simulink model "playback_data_4"  (R2015a)
settings: Solver=FixedStepDiscrete  SolverMode=SingleTasking  StartTime=0  StopTime=time_recorded(end)  FixedStep=sample_time  RelTol=1e-3
undefined symbols (not defined in the file): A1_notch_f1, A2_notch_f1, A_kalman_transverse, A_kalman_vertical, A_lpf_dtau, A_lpf_fourbar_angles, A_lpf_imu, A_lpf_lateral_angle, A_lpf_leg_spring, B1_lpf_dtau, B1_lpf_fourbar_angles, B1_lpf_imu, B1_lpf_lateral_angle, B1_lpf_leg_spring, B1_notch_f1, B2_lpf_dtau, B2_lpf_fourbar_angles, B2_lpf_imu, B2_lpf_lateral_angle, B2_lpf_leg_spring, B2_notch_f1, B_dx_versus_x0, B_kalman_transverse, B_kalman_vertical, backwards_K_front_of_t_row1, backwards_K_front_of_t_row2, backwards_K_sag_of_t, backwards_P_front_of_t, backwards_P_sag_of_t, C_kalman_transverse, C_kalman_vertical, com_leg_motor, com_torso, contact_threshold, control_start_time, d_ankle_to_foot, d_vertical_com, desired_com_forward_velocity, desired_com_lateral_velocity, desired_initial_leg_roll_left, desired_initial_leg_roll_right, desired_lateral_symmetry_angle, desired_standing_torso_pitch, desired_standing_torso_roll, desired_standing_z, desired_torso_pitch, desired_torso_roll, Discrete, fcut_contact, forward_dx_of_dxstar, forward_x_of_dxstar, g, gain_nodes_sea_torque, HIP_MTR_MAX_CONT_TORQUE, HIP_MTR_MAX_TORQUE, i_leg_motor, i_robot, i_torso, initial_dx_estimate, initial_dy_estimate ... (+75)
libraries: simulink x12, ctrlSharedLib x3
(part 3 of 5)

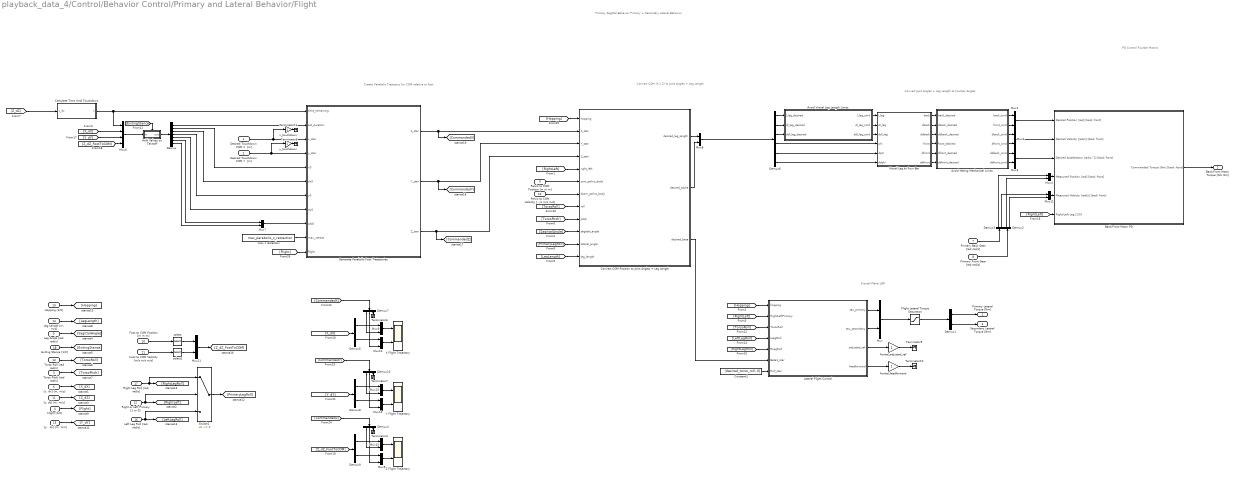
== system playback_data_4/Control/Behavior Control/Primary and Lateral Behavior/Flight ==
  note: Frontal Plane LQR
  note: PD Control Fourbar Motors
  note: Convert Joint Angles + Leg Length
      | to Fourbar Angles
  note: Convert COM (X,Y,Z) to
      | Joint Angles + Leg Length
  note: Create Parabolic
      | Trajectory for COM relative to foot
  note: Primary Sagittal Behavior
      | Primary + Secondary Lateral Behavior
  Desired Touchdown COM X  [m] : Inport
  Desired Touchdown COM Y  [m] : Inport  Port=2
  Torso Pitch [rad rad/s] : Inport  Port=3
  Flight [1/0] : Inport  Port=4
  Leg Angle [rad rad/s] : Inport  Port=5
  "[x, dx] [m, m/s]" : Inport  Port=6
  Primary Back Gear [rad rad/s] : Inport  Port=7
  Primary Front Gear [rad rad/s] : Inport  Port=8
  Pelvis to COM Position [m m m] : Inport  Port=9
  Pelvis to COM Velocity [m/s m/s m/s] : Inport  Port=10
  "[z, dz] [m, m/s]" : Inport  Port=11
  Right or Left Primary [1 or 0] : Inport  Port=12
  Torso Roll [rad rad/s] : Inport  Port=13
  "Leg Length [m, m/s]" : Inport  Port=14
  "[y,  dy] [m, m/s]" : Inport  Port=15
  "Left Leg Roll [rad, rad/s]" : Inport  Port=16
  "Right Leg Roll [rad, rad/s]" : Inport  Port=17
  Exiting Stance [1/0] : Inport  Port=18
  Hopping [1/0] : Inport  Port=19
  Foot to COM Position [m m m] : Inport  Port=20
  Foot to COM Velocity [m/s m/s m/s] : Inport  Port=21
  Avoid Hitting Mechanical Limits : MATLAB Function  TreatAsAtomicUnit=on
  Avoid Virtual Leg Length Limits : MATLAB Function  TreatAsAtomicUnit=on
  Back/Front Motor PD : Subsystem
  Calculate Time Until Touchdown : MATLAB Function  TreatAsAtomicUnit=on
  Constant1 : Constant  Value=[desired_torso_roll; 0]
  "Convert COM Position to Joint Angles + Leg Length " : MATLAB Function  TreatAsAtomicUnit=on
  Demux : Demux  Outputs=7
  Demux{1..3,5,8..9} (6 alike) : Demux  Outputs=2
  Demux10 : Demux  Outputs=3
  Demux4 : Demux  Outputs=3
  Demux6 : Demux  Outputs=6
  Demux7 : Demux  Outputs=3
  Flight Lateral Torque Saturation : Saturate  UpperLimit=HIP_MTR_MAX_CONT_TORQUE  LowerLimit=-HIP_MTR_MAX_CONT_TORQUE
      settings: AttributesFormatString=Top: %<UpperLimit>\nBottom: %<LowerLimit>
  Generate Parabolic Foot Trajectories : MATLAB Function  TreatAsAtomicUnit=on
  Hold Values on Takeoff : Subsystem
  Lateral Flight Control : MATLAB Function  TreatAsAtomicUnit=on
  Mux{,1..5,7..13,15,21} (15 alike) : Mux  Inputs=2
  Mux6 : Mux
  Switch1 : Switch  Criteria=u2 ~= 0
  Terminator{4..7,9..11} (7 alike) : Terminator
  Virtual Leg to Four Bar : MATLAB Function  TreatAsAtomicUnit=on
  X Flight Trajectory : Scope  NumInputPorts=2
      settings: YMin=-1~-0.8  YMax=1~1.4  SaveName=ScopeData3  SampleInput=on
  Y Flight Trajectory : Scope  NumInputPorts=2
      settings: YMin=-1~-0.8  YMax=1~1.4  SaveName=ScopeData4  SampleInput=on
  Z Flight Trajectory : Scope  NumInputPorts=2
      settings: YMin=-1~-0.8  YMax=1~1.4  SaveName=ScopeData7  SampleInput=on
  frontal_adjusted_ref : Gain
  frontal_feedforward : Gain
  max z retraction : Constant  Value=max_parabolic_z_retraction
  select : Selector  InputPortWidth=3  Indices=[3]
  select1 : Selector  InputPortWidth=3  Indices=[3]
  x_touchdown : Gain
  y_touchdown : Gain
  Back/Front Motor Torque [Nm Nm] : Outport
  Primary Lateral Torque [Nm] : Outport  Port=2
  Secondary Lateral Torque [Nm] : Outport  Port=3
  wires:
  Generate Parabolic Foot Trajectories/3(Z_star) -> [CommandedZ], "Convert COM Position to Joint Angles + Leg Length "/4(Z_star)
  [CommandedZ] -> Demux4/1
  [CommandedY] -> Demux10/1
  [CommandedX] -> Demux7/1
  Demux10/3 -> Terminator7/1
  [Y_dY] -> Demux8/1
  Demux10/2 -> Mux12/2
  Demux10/1 -> Mux13/2
  Demux8/2 -> Mux12/1
  Demux8/1 -> Mux13/1
  Mux12/1 -> Y Flight Trajectory/2
  Mux13/1 -> Y Flight Trajectory/1
  Demux7/3 -> Terminator6/1
  [X_dX] -> Demux5/1
  Demux7/2 -> Mux10/2
  Demux7/1 -> Mux9/2
  Demux5/2 -> Mux10/1
  Demux5/1 -> Mux9/1
  Mux10/1 -> X Flight Trajectory/2
  Mux9/1 -> X Flight Trajectory/1
  Demux4/3 -> Terminator4/1
  Demux4/2 -> Mux5/2
  Demux4/1 -> Mux15/2
  Demux9/2 -> Mux5/1
  Demux9/1 -> Mux15/1
  [Z_dZ_FootToCOM] -> Demux9/1
  [Z_dZ_FootToCOM] -> Mux6/4
  Mux5/1 -> Z Flight Trajectory/2
  Mux15/1 -> Z Flight Trajectory/1
  Mux21/1 -> [Z_dZ_FootToCOM]
  select1/1 -> Mux21/2
  select/1 -> Mux21/1
  Foot to COM Velocity [m/s m/s m/s]/1 -> select1/1
  Foot to COM Position [m m m]/1 -> select/1
  Demux/7 -> Mux7/2
  Demux/6 -> Mux7/1
  Demux/5 -> Generate Parabolic Foot Trajectories/8(dy0)
  Demux/4 -> Generate Parabolic Foot Trajectories/7(y0)
  Demux/3 -> Generate Parabolic Foot Trajectories/6(dx0)
  Demux/2 -> Generate Parabolic Foot Trajectories/5(x0)
  [Flight] -> Generate Parabolic Foot Trajectories/11(flight)
  Hopping [1/0]/1 -> [Hopping]
  [Hopping] -> Lateral Flight Control/1(hopping)
  Mux/1 -> Flight Lateral Torque Saturation/1
  [Hopping] -> "Convert COM Position to Joint Angles + Leg Length "/1(hopping)
  frontal_adjusted_ref/1 -> Terminator9/1
  frontal_feedforward/1 -> Terminator10/1
  Flight Lateral Torque Saturation/1 -> Demux1/1
  "Convert COM Position to Joint Angles + Leg Length "/3(desired_beta) -> Lateral Flight Control/6(Beta1_star)
  Demux1/2 -> Secondary Lateral Torque [Nm]/1
  Demux1/1 -> Primary Lateral Torque [Nm]/1
  Exiting Stance [1/0]/1 -> [ExitingStance]
  Switch1/1 -> [PrimaryLegRoll]
  Right or Left Primary [1 or 0]/1 -> [RightLeft], Switch1/2
  "Right Leg Roll [rad, rad/s]"/1 -> [RightLegRoll], Switch1/1
  [RightLegRoll] -> Lateral Flight Control/5(RLegRoll)
  [LeftLegRoll] -> Lateral Flight Control/4(LLegRoll)
  "Left Leg Roll [rad, rad/s]"/1 -> [LeftLegRoll], Switch1/3
  Lateral Flight Control/1(tau_primary) -> Mux/1
  Lateral Flight Control/2(tau_secondary) -> Mux/2
  Lateral Flight Control/4(feedforward) -> frontal_feedforward/1
  Lateral Flight Control/3(adjusted_ref) -> frontal_adjusted_ref/1
  Constant1/1 -> Lateral Flight Control/7(Roll_star)
  [TorsoRoll] -> Lateral Flight Control/3(TorsoRoll)
  [RightLeft] -> Lateral Flight Control/2(RightLeftPrimary)
  Desired Touchdown COM Y  [m]/1 -> Generate Parabolic Foot Trajectories/4(y_star), y_touchdown/1
  Demux6/3 -> Avoid Virtual Leg Length Limits/3(ddl_leg_desired)
  Demux6/2 -> Avoid Virtual Leg Length Limits/2(dl_leg_desired)
  Demux6/1 -> Avoid Virtual Leg Length Limits/1(l_leg_desired)
  Avoid Virtual Leg Length Limits/3(ddl_leg_cmd) -> Virtual Leg to Four Bar/3(ddl_leg)
  Avoid Virtual Leg Length Limits/2(dl_leg_cmd) -> Virtual Leg to Four Bar/2(dl_leg)
  Avoid Virtual Leg Length Limits/1(l_leg_cmd) -> Virtual Leg to Four Bar/1(l_leg)
  Calculate Time Until Touchdown/1(t) -> Generate Parabolic Foot Trajectories/1(time_remaining), Mux6/1
  [Z_dZ] -> Calculate Time Until Touchdown/1(z_dz)
  [Y_dY] -> Mux6/3
  "[y,  dy] [m, m/s]"/1 -> [Y_dY]
  y_touchdown/1 -> Terminator5/1
  x_touchdown/1 -> Terminator11/1
  Desired Touchdown COM X  [m]/1 -> x_touchdown/1, Generate Parabolic Foot Trajectories/3(x_star)
  "[z, dz] [m, m/s]"/1 -> [Z_dZ]
  "Leg Length [m, m/s]"/1 -> [LegLength]
  Torso Roll [rad rad/s]/1 -> [TorsoRoll]
  "[x, dx] [m, m/s]"/1 -> [X_dX]
  [ExitingStance] -> Hold Values on Takeoff/Trigger
  Flight [1/0]/1 -> [Flight]
  Pelvis to COM Velocity [m/s m/s m/s]/1 -> "Convert COM Position to Joint Angles + Leg Length "/7(dcom_pelvis_body)
  Pelvis to COM Position [m m m]/1 -> "Convert COM Position to Joint Angles + Leg Length "/6(com_pelvis_body)
  [TorsoRoll] -> "Convert COM Position to Joint Angles + Leg Length "/8(roll)
  [LegLength] -> "Convert COM Position to Joint Angles + Leg Length "/12(leg_length)
  [PrimaryLegRoll] -> "Convert COM Position to Joint Angles + Leg Length "/11(lateral_angle)
  [TorsoPitch] -> "Convert COM Position to Joint Angles + Leg Length "/9(pitch)
  Torso Pitch [rad rad/s]/1 -> [TorsoPitch]
  [SagittalAngle] -> "Convert COM Position to Joint Angles + Leg Length "/10(sagittal_angle)
  Leg Angle [rad rad/s]/1 -> [SagittalAngle]
  Mux8/1 -> Demux6/1
  Demux6/4 -> Virtual Leg to Four Bar/4(phi)
  Demux6/5 -> Virtual Leg to Four Bar/5(dphi)
  Demux6/6 -> Virtual Leg to Four Bar/6(ddphi)
  "Convert COM Position to Joint Angles + Leg Length "/1(desired_leg_length) -> Mux8/1
  "Convert COM Position to Joint Angles + Leg Length "/2(desired_alpha) -> Mux8/2
  [RightLeft] -> "Convert COM Position to Joint Angles + Leg Length "/5(right_left)
  Generate Parabolic Foot Trajectories/2(Y_star) -> [CommandedY], "Convert COM Position to Joint Angles + Leg Length "/3(Y_star)
  Generate Parabolic Foot Trajectories/1(X_star) -> "Convert COM Position to Joint Angles + Leg Length "/2(X_star), [CommandedX]
  [X_dX] -> Mux6/2
  Hold Values on Takeoff/1(out) -> Demux/1
  Mux6/1 -> Hold Values on Takeoff/1(in)
  max z retraction/1 -> Generate Parabolic Foot Trajectories/10(max_retract)
  Mux7/1 -> Generate Parabolic Foot Trajectories/9(zdz0)
  Demux/1 -> Generate Parabolic Foot Trajectories/2(est_duration)
  [RightLeft] -> Back/Front Motor PD/6(Right/Left Leg [1/0])
  Primary Front Gear [rad rad/s]/1 -> Demux2/1
  Primary Back Gear [rad rad/s]/1 -> Demux3/1
  Back/Front Motor PD/1(Commanded Torque [Nm] [back front]) -> Back/Front Motor Torque [Nm Nm]/1
  Mux3/1 -> Back/Front Motor PD/3(Desired Acceleration [rad/s^2] [back front])
  Mux2/1 -> Back/Front Motor PD/2(Desired Velocity [rad/s] [back front])
  Avoid Hitting Mechanical Limits/6(ddfront_cmd) -> Mux3/2
  Avoid Hitting Mechanical Limits/5(ddback_cmd) -> Mux3/1
  Avoid Hitting Mechanical Limits/4(dfront_cmd) -> Mux2/2
  Avoid Hitting Mechanical Limits/3(dback_cmd) -> Mux2/1
  Demux2/1 -> Mux4/2
  Avoid Hitting Mechanical Limits/1(back_cmd) -> Mux1/1
  Avoid Hitting Mechanical Limits/2(front_cmd) -> Mux1/2
  Demux3/1 -> Mux4/1
  Demux3/2 -> Mux11/1
  Mux1/1 -> Back/Front Motor PD/1(Desired Position [rad] [back front])
  Mux4/1 -> Back/Front Motor PD/4(Measured Position [rad] [back front])
  Demux2/2 -> Mux11/2
  Mux11/1 -> Back/Front Motor PD/5(Measured Velocity [rad/s] [back front])
  Virtual Leg to Four Bar/6(ddfront) -> Avoid Hitting Mechanical Limits/6(ddfront_desired)
  Virtual Leg to Four Bar/5(dfront) -> Avoid Hitting Mechanical Limits/5(dfront_desired)
  Virtual Leg to Four Bar/4(front) -> Avoid Hitting Mechanical Limits/4(front_desired)
  Virtual Leg to Four Bar/3(ddback) -> Avoid Hitting Mechanical Limits/3(ddback_desired)
  Virtual Leg to Four Bar/2(dback) -> Avoid Hitting Mechanical Limits/2(dback_desired)
  Virtual Leg to Four Bar/1(back) -> Avoid Hitting Mechanical Limits/1(back_desired)

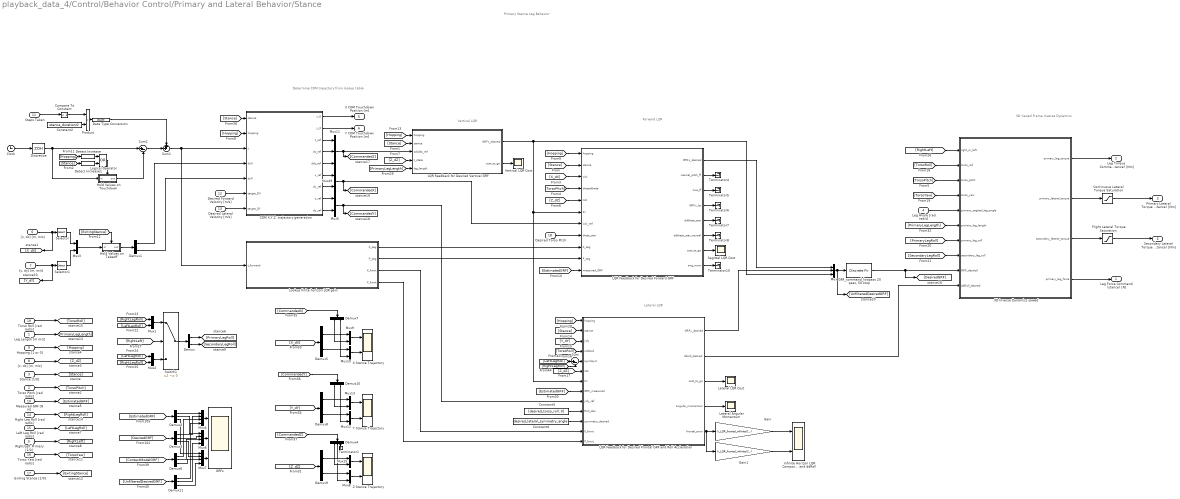
== system playback_data_4/Control/Behavior Control/Primary and Lateral Behavior/Stance ==
  note: Lateral LQR
  note: 3D Yawed Frame Inverse Dynamics
  note: Forward LQR
  note: Vertical LQR
  note: Determine COM trajectory
      | from lookup table
  note: Primary Stance Leg Behavior
  Leg Length [m m/s] : Inport
  Torso Pitch [rad rad/s] : Inport  Port=2
  Stance [1/0] : Inport  Port=3
  Leg Angle [rad rad/s] : Inport  Port=4
  Right/Left Primary [1/0] : Inport  Port=5
  "[x, dx] [m, m/s]" : Inport  Port=6
  "[y, dy] [m, m/s]" : Inport  Port=7
  "[z, dz] [m, m/s]" : Inport  Port=8
  Hopping [1 or 0] : Inport  Port=9
  Measured GRF [N N] : Inport  Port=10
  Steps Taken : Inport  Port=11
  Desired Forward Velocity [m/s] : Inport  Port=12
  Desired Lateral Velocity [m/s] : Inport  Port=13
  Right Leg Roll [rad rad/s] : Inport  Port=14
  Left Leg Roll [rad rad/s] : Inport  Port=15
  Torso Yaw [rad rad/s] : Inport  Port=16
  Exiting Stance [1/0] : Inport  Port=17
  Desired Torso Pitch : Inport  Port=18
  Torso Roll [rad rad/s] : Inport  Port=19
  3D Inverse Dynamics yawed : MATLAB Function  TreatAsAtomicUnit=on
  COM X,Y,Z  trajectory generation : MATLAB Function  TreatAsAtomicUnit=on
  Clock : Clock
  Compare To Constant : simulink/Logic and Bit Operations/Compare To Constant  relop=<  const=1  OutDataTypeStr=uint8
  Constant2 : Constant  Value=stance_duration/2
  Constant5 : Constant  Value=[desired_torso_roll; 0]
  Constant6 : Constant  Value=desired_lateral_symmetry_angle
  Continuous Lateral Torque Saturation : Saturate  UpperLimit=HIP_MTR_MAX_CONT_TORQUE  LowerLimit=-HIP_MTR_MAX_CONT_TORQUE
      settings: AttributesFormatString=Top: %<UpperLimit>\nBottom: %<LowerLimit>
  Data Type Conversion : DataTypeConversion  OutDataTypeStr=double
  Demux{,1,5,7..10} (7 alike) : Demux  Outputs=2
  Demux{2..4,6,11} (5 alike) : Demux  Outputs=3
  Detect Increase : simulink/Logic and Bit Operations/Detect Increase  vinit=0.0  InputProcessing=Inherited  OutDataTypeStr=boolean
  Detect Increase1 : simulink/Logic and Bit Operations/Detect Increase  vinit=0.0  InputProcessing=Inherited  OutDataTypeStr=boolean
  Discretize : ZeroOrderHold  SampleTime=sample_time
  Flight Lateral Torque Saturation : Saturate  UpperLimit=HIP_MTR_MAX_CONT_TORQUE  LowerLimit=-HIP_MTR_MAX_CONT_TORQUE
      settings: AttributesFormatString=Top: %<UpperLimit>\nBottom: %<LowerLimit>
  "GRF_command_lowpass 20 pass, 50 stop" : DiscreteFir  Tag=BlockMethodSubSystem  Coefficients=[-0.0065303670489285049 -0.0039313926403470242 -0.0048630776000435465 -0.0057248908722514107 -0.0064402270401543553 -0.0069124881718239713 -0.0070550751837271126 -0.0067763964248262719 -0.0059955884962007702 -0.0046203515932795149 -0.0026164712407433744 5.5625054243875136e-05 0.0034168828763037565 0.0074322120212943236 0.012066519706809652 0.01722807163822164 0.022817702983514012 0.028694941256765513 0.03470395198526529 0.040669941556379492 0.046421058403681451 0.051764290707578361 0.056533861311620921 0.060562831216546612 0.063716802641316989 0.06588388946005809 0.066985417581438667 0.066985417581438667 0.06588388946005809 0.063716802641316989 0.060562831216546612 0.056533861311620921 0.051764290707578361 0.046421058403681451 0.040669941556379492 0.03470395198526529 0.028694941256765513 0.022817702983514012 0.01722807163822164 0.012066519706809652 0.0074322120212943236 0.0034168828763037565 5.5625054243875136e-05 -0.0026164712407433744 -0.0046203515932795149 -0.0059955884962007702 -0.0067763964248262719 -0.0070550751837271126 -0.0069124881718239713 -0.0064402270401543553 -0.0057248908722514107 -0.0048630776000435465 -0.0039313926403470242 -0.0065303670489285049]  SampleTime=sample_time
  GRFs : Scope  NumInputPorts=3
      settings: TimeRange=0.3720061688053303  YMin=-12.5~-40~0  YMax=15~80~4000  SampleInput=on
  Gain : Gain  Gain=k_LQR_frontal_infinite(1,:)
  Gain1 : Gain  Gain=k_LQR_frontal_infinite(2,:)
  Hold Values on Takeoff : Subsystem
  Hold Values on Touchdown : Subsystem
  "Infinite Horizon LQR Components y, roll, sym, dy, droll, L GRFy and ddRoll" : Scope  NumInputPorts=2
      settings: YMin=-3.5~-5  YMax=4~5  SaveName=ScopeData12  SampleInput=on
  LQR Feedback for Desired Forward GRF : MATLAB Function  TreatAsAtomicUnit=on
  LQR Feedback for Desired Frontal GRF and Roll Accleration : MATLAB Function  TreatAsAtomicUnit=on
  LQR Feedback for Desired Vertical GRF : MATLAB Function  TreatAsAtomicUnit=on
  Lateral Angular Momentum : Scope
      settings: YMin=-3.5  YMax=4  SaveName=ScopeData20  SampleInput=on
  Lateral LQR Cost : Scope
      settings: YMin=100  YMax=240  SaveName=ScopeData9  SampleInput=on
  Logical Operator : Logic  Operator=OR  AllPortsSameDT=off  OutDataTypeStr=boolean
  Lookup finite horizon LQR gain : MATLAB Function  TreatAsAtomicUnit=on
  Mux : Mux  Inputs=3
  Mux{1..3,5,8..10,12..13,15,49} (11 alike) : Mux  Inputs=2
  Mux11 : Mux  Inputs=3
  Mux4 : Mux
  Mux6 : Mux
  Mux7 : Mux
  Product : Product
  Sagittal LQR Cost : Scope
      settings: YMin=22.5  YMax=62.5  SaveName=ScopeData10  SampleInput=on
  Selector : Selector  InputPortWidth=2  Indices=[2]
  Selector1 : Selector  InputPortWidth=2  Indices=[2]
  Sum : Sum  Inputs=|+-
  Sum1 : Sum  Inputs=++|  OutDataTypeStr=double
  Sum2 : Sum  Inputs=|+-
  Switch1 : Switch  Criteria=u2 ~= 0
  Terminator{1,4..8,10} (7 alike) : Terminator
  Vertical LQR Cost : Scope
      settings: YMin=11  YMax=16  SaveName=ScopeData18  SampleInput=on
  X Stance Trajectory : Scope  NumInputPorts=2
      settings: YMin=0~-0.02  YMax=0.005~0.03  SaveName=ScopeData8  SampleInput=on
  Y Stance Trajectory : Scope  NumInputPorts=2
      settings: YMin=0.005~-0.5  YMax=0.1~0.3  SaveName=ScopeData5  SampleInput=on
  Z Stance Trajectory : Scope  NumInputPorts=2
      settings: YMin=0~-1.25  YMax=1.05~1.5  SaveName=ScopeData6  SampleInput=on
  Leg Force Command (stance) [N] : Outport
  Leg Torque Command (stance) [Nm] : Outport  Port=2
  Primary Lateral Torque Command (stance) [Nm] : Outport  Port=3
  Secondary Lateral Torque Command (stance) [Nm] : Outport  Port=4
  X COM Touchdown Position [m] : Outport  Port=5
  Y COM Touchdown Position [m] : Outport  Port=6
  wires:
  Gain1/1 -> "Infinite Horizon LQR Components y, roll, sym, dy, droll, L GRFy and ddRoll"/2
  LQR Feedback for Desired Frontal GRF and Roll Accleration/5(frontal_error) -> Gain/1, Gain1/1
  Gain/1 -> "Infinite Horizon LQR Components y, roll, sym, dy, droll, L GRFy and ddRoll"/1
  Continuous Lateral Torque Saturation/1 -> Primary Lateral Torque Command (stance) [Nm]/1
  3D Inverse Dynamics yawed/3(secondary_lateral_torque) -> Flight Lateral Torque Saturation/1
  3D Inverse Dynamics yawed/2(primary_lateral_torque) -> Continuous Lateral Torque Saturation/1
  Demux11/3 -> Mux7/4
  Demux11/2 -> Mux6/4
  Demux11/1 -> Mux4/4
  [UnfilteredDesiredGRF] -> Demux11/1
  "GRF_command_lowpass 20 pass, 50 stop"/1 -> [DesiredGRF], 3D Inverse Dynamics yawed/9(GRF_desired)
  LQR Feedback for Desired Forward GRF/1(GRFx_desired) -> Mux/1
  Left Leg Roll [rad rad/s]/1 -> [LeftLegRoll]
  Right/Left Primary [1/0]/1 -> [RightLeft]
  [CommandedZ] -> Demux4/1
  [CommandedY] -> Demux10/1
  [CommandedX] -> Demux7/1
  [Y_dY] -> Demux8/1
  Demux10/2 -> Mux12/2
  Demux10/1 -> Mux13/2
  Demux8/2 -> Mux12/1
  Demux8/1 -> Mux13/1
  Mux12/1 -> Y Stance Trajectory/2
  Mux13/1 -> Y Stance Trajectory/1
  [X_dX] -> Demux5/1
  Demux7/2 -> Mux10/2
  Demux7/1 -> Mux9/2
  Demux5/2 -> Mux10/1
  Demux5/1 -> Mux9/1
  Mux10/1 -> X Stance Trajectory/2
  Mux9/1 -> X Stance Trajectory/1
  Demux4/3 -> Terminator1/1
  Demux4/2 -> Mux8/2
  Demux4/1 -> Mux15/2
  Demux9/2 -> Mux8/1
  Demux9/1 -> Mux15/1
  [Z_dZ] -> Demux9/1
  Mux8/1 -> Z Stance Trajectory/2
  Mux15/1 -> Z Stance Trajectory/1
  Demux3/3 -> Mux7/2
  Demux3/2 -> Mux6/2
  Demux3/1 -> Mux4/2
  Demux2/3 -> Mux7/1
  Demux2/2 -> Mux6/1
  Mux7/1 -> GRFs/3
  Mux6/1 -> GRFs/2
  Demux2/1 -> Mux4/1
  Mux4/1 -> GRFs/1
  [DesiredGRF] -> Demux3/1
  [EstimatedGRF] -> Demux2/1
  Torso Roll [rad rad/s]/1 -> [TorsoRoll]
  [PrimaryLegLength] -> LQR Feedback for Desired Vertical GRF/5(leg_length)
  Leg Length [m m/s]/1 -> [PrimaryLegLength]
  Discretize/1 -> Sum2/1, Hold Values on Touchdown/1(in)
  [EstimatedGRF] -> LQR Feedback for Desired Frontal GRF and Roll Accleration/8(GRF_measured)
  [Hopping] -> LQR Feedback for Desired Frontal GRF and Roll Accleration/1(hopping)
  3D Inverse Dynamics yawed/4(primary_leg_force) -> Leg Force Command (stance) [N]/1
  [ExitingStance] -> Hold Values on Takeoff/Trigger
  Exiting Stance [1/0]/1 -> [ExitingStance]
  Torso Yaw [rad rad/s]/1 -> [TorsoYaw]
  Desired Lateral Velocity [m/s]/1 -> COM X,Y,Z  trajectory generation/7(target_DY)
  Selector1/1 -> Mux3/2
  Hold Values on Takeoff/1(out) -> Demux1/1
  Mux3/1 -> Hold Values on Takeoff/1(in)
  "[y, dy] [m, m/s]"/1 -> Selector1/1, [Y_dY]
  [RightLeft] -> Switch1/2
  [RightLegRoll] -> Mux2/2
  [LeftLegRoll] -> Mux2/1
  [LeftLegRoll] -> Mux1/2
  [RightLegRoll] -> Mux1/1
  Right Leg Roll [rad rad/s]/1 -> [RightLegRoll]
  Mux2/1 -> Switch1/3
  Mux1/1 -> Switch1/1
  Demux/1 -> [PrimaryLegRoll]
  Demux/2 -> [SecondaryLegRoll]
  Switch1/1 -> Demux/1
  [PrimaryLegRoll] -> 3D Inverse Dynamics yawed/7(primary_leg_roll)
  [SecondaryLegRoll] -> 3D Inverse Dynamics yawed/8(secondary_leg_roll)
  Leg Angle [rad rad/s]/1 -> 3D Inverse Dynamics yawed/5(primary_sagittal_leg_angle)
  [PrimaryLegLength] -> 3D Inverse Dynamics yawed/6(primary_leg_length)
  [TorsoYaw] -> 3D Inverse Dynamics yawed/4(torso_yaw)
  [TorsoRoll] -> 3D Inverse Dynamics yawed/2(torso_roll)
  [TorsoPitch] -> 3D Inverse Dynamics yawed/3(torso_pitch)
  Mux/1 -> "GRF_command_lowpass 20 pass, 50 stop"/1, [UnfilteredDesiredGRF]
  Mux5/1 -> LQR Feedback for Desired Frontal GRF and Roll Accleration/9(ydy_ref), [CommandedY]
  COM X,Y,Z  trajectory generation/2(y_0) -> Y COM Touchdown Position [m]/1
  Sum/1 -> LQR Feedback for Desired Frontal GRF and Roll Accleration/5(symdsym)
  [LeftLegRoll] -> Sum/1
  [RightLegRoll] -> Sum/2
  [Z_dZ] -> LQR Feedback for Desired Frontal GRF and Roll Accleration/6(zdz)
  [TorsoRoll] -> LQR Feedback for Desired Frontal GRF and Roll Accleration/4(rolldroll)
  [Y_dY] -> LQR Feedback for Desired Frontal GRF and Roll Accleration/3(ydy)
  [Stance] -> LQR Feedback for Desired Frontal GRF and Roll Accleration/2(stance)
  LQR Feedback for Desired Frontal GRF and Roll Accleration/1(GRFy_desired) -> Mux/2
  LQR Feedback for Desired Frontal GRF and Roll Accleration/2(ddroll_desired) -> 3D Inverse Dynamics yawed/10(ddRoll_desired)
  LQR Feedback for Desired Frontal GRF and Roll Accleration/3(cost_to_go) -> Lateral LQR Cost/1
  Lookup finite horizon LQR gain/3(K_front) -> LQR Feedback for Desired Frontal GRF and Roll Accleration/12(K_front)
  Constant5/1 -> LQR Feedback for Desired Frontal GRF and Roll Accleration/10(Roll_star)
  Constant6/1 -> LQR Feedback for Desired Frontal GRF and Roll Accleration/11(symmetry_desired)
  [Hopping] -> LQR Feedback for Desired Vertical GRF/1(hopping)
  Selector/1 -> Mux3/1
  Demux1/1 -> COM X,Y,Z  trajectory generation/4(dx0)
  [Stance] -> Detect Increase1/1
  [Hopping] -> Detect Increase/1
  Data Type Conversion/1 -> Sum1/1
  Sum2/1 -> Sum1/2
  Compare To Constant/1 -> Product/1
  Detect Increase1/1 -> Logical Operator/2
  Detect Increase/1 -> Logical Operator/1
  Constant2/1 -> Product/2
  Product/1 -> Data Type Conversion/1
  Steps Taken/1 -> Compare To Constant/1
  [EstimatedGRF] -> LQR Feedback for Desired Forward GRF/11(measured_GRF)
  Measured GRF [N N]/1 -> [EstimatedGRF]
  [Hopping] -> LQR Feedback for Desired Forward GRF/1(hopping)
  [Hopping] -> COM X,Y,Z  trajectory generation/2(hopping)
  Hopping [1 or 0]/1 -> [Hopping]
  [RightLeft] -> 3D Inverse Dynamics yawed/1(right_or_left)
  Torso Pitch [rad rad/s]/1 -> [TorsoPitch]
  LQR Feedback for Desired Forward GRF/8(ang_mom) -> Terminator10/1
  LQR Feedback for Desired Forward GRF/7(cost_to_go) -> Sagittal LQR Cost/1
  LQR Feedback for Desired Forward GRF/6(ddtheta_star_neutral) -> Terminator8/1
  LQR Feedback for Desired Forward GRF/5(ddtheta_star) -> Terminator7/1
  LQR Feedback for Desired Forward GRF/3(true_ff) -> Terminator5/1
  LQR Feedback for Desired Forward GRF/2(netural_pitch_ff) -> Terminator4/1
  LQR Feedback for Desired Vertical GRF/2(cost_to_go) -> Vertical LQR Cost/1
  Demux1/2 -> COM X,Y,Z  trajectory generation/5(dy0)
  Clock/1 -> Discretize/1
  "[x, dx] [m, m/s]"/1 -> Selector/1, [X_dX]
  Logical Operator/1 -> Hold Values on Touchdown/Trigger
  [Stance] -> LQR Feedback for Desired Vertical GRF/2(stance)
  Stance [1/0]/1 -> [Stance]
  Hold Values on Touchdown/1(out) -> Sum2/2
  LQR Feedback for Desired Vertical GRF/1(GRFz_desired) -> Mux/3, LQR Feedback for Desired Forward GRF/6(Fz), LQR Feedback for Desired Frontal GRF and Roll Accleration/7(Fz)
  Sum1/1 -> COM X,Y,Z  trajectory generation/3(t), Lookup finite horizon LQR gain/1(t_forward)
  Desired Forward Velocity [m/s]/1 -> COM X,Y,Z  trajectory generation/6(target_DX)
  [Z_dZ] -> LQR Feedback for Desired Forward GRF/5(zdz)
  Lookup finite horizon LQR gain/1(K_sag) -> LQR Feedback for Desired Forward GRF/9(K_sag)
  Desired Torso Pitch/1 -> LQR Feedback for Desired Forward GRF/8(theta_star)
  Mux49/1 -> LQR Feedback for Desired Forward GRF/7(xdx_ref), [CommandedX]
  [TorsoPitch] -> LQR Feedback for Desired Forward GRF/4(thetadtheta)
  [X_dX] -> LQR Feedback for Desired Forward GRF/3(xdx)
  Mux11/1 -> LQR Feedback for Desired Vertical GRF/3(zdzddz_ref), [CommandedZ]
  COM X,Y,Z  trajectory generation/5(ddz_ref) -> Mux11/3
  COM X,Y,Z  trajectory generation/4(dz_ref) -> Mux11/2
  COM X,Y,Z  trajectory generation/1(x_0) -> X COM Touchdown Position [m]/1
  COM X,Y,Z  trajectory generation/9(dy_ref) -> Mux5/2
  COM X,Y,Z  trajectory generation/8(y_ref) -> Mux5/1
  COM X,Y,Z  trajectory generation/7(dx_ref) -> Mux49/2
  COM X,Y,Z  trajectory generation/6(x_ref) -> Mux49/1
  [Stance] -> LQR Feedback for Desired Forward GRF/2(stance)
  COM X,Y,Z  trajectory generation/3(z_ref) -> Mux11/1
  [Z_dZ] -> LQR Feedback for Desired Vertical GRF/4(z_state)
  3D Inverse Dynamics yawed/1(primary_leg_torque) -> Leg Torque Command (stance) [Nm]/1
  Lookup finite horizon LQR gain/2(P_sag) -> LQR Feedback for Desired Forward GRF/10(P_sag)
  Lookup finite horizon LQR gain/4(P_front) -> LQR Feedback for Desired Frontal GRF and Roll Accleration/13(P_front)
  [Stance] -> COM X,Y,Z  trajectory generation/1(stance)
  LQR Feedback for Desired Forward GRF/4(GRFx_lqr) -> Terminator6/1
  LQR Feedback for Desired Frontal GRF and Roll Accleration/4(angular_momentum) -> Lateral Angular Momentum/1
  [ContactModelGRF] -> Demux6/1
  Demux6/1 -> Mux4/3
  Demux6/2 -> Mux6/3
  Demux6/3 -> Mux7/3
  Flight Lateral Torque Saturation/1 -> Secondary Lateral Torque Command (stance) [Nm]/1
  "[z, dz] [m, m/s]"/1 -> [Z_dZ]

== system playback_data_4/Control/Behavior Control/Secondary Leg Behavior/Back//Front Motor PD ==
  Desired Position [rad] [back front] : Inport
  Desired Velocity [rad/s] [back front] : Inport  Port=2
  Desired Acceleration [rad/s^2] [back front] : Inport  Port=3
  Measured Position [rad] [back front] : Inport  Port=4
  Measured Velocity [rad/s] [back front] : Inport  Port=5
  Right/Left Leg [1/0] : Inport  Port=6
  Divide : Product  Inputs=*/
  Friction Compensation : Subsystem
  Load Torque in Flight : Constant  Value=30
  Motor Efficiency : MATLAB Function  TreatAsAtomicUnit=on
  Product : Product
  RPM in Flight : Constant  Value=0
  Sum1 : Sum  Inputs=|++
  Sum2 : Sum  Inputs=|++
  Sum7 : Sum  Inputs=|+-
  Sum8 : Sum  Inputs=|+-
  Sum9 : Sum
  kd : Gain  Gain=kd_motor
  kp : Gain  Gain=kp_motor
  reflected inertia : Constant  Value=j_motor
  Commanded Torque [Nm] [back front] : Outport
  wires:
  Load Torque in Flight/1 -> Motor Efficiency/2(load_torque)
  Sum1/1 -> Divide/1
  Divide/1 -> Sum2/1
  Motor Efficiency/1(mu) -> Divide/2
  RPM in Flight/1 -> Motor Efficiency/1(rpm)
  reflected inertia/1 -> Product/2
  Desired Velocity [rad/s] [back front]/1 -> Sum8/1, Friction Compensation/2(Commanded Velocity [rad/s] [back front])
  Sum2/1 -> Commanded Torque [Nm] [back front]/1
  Right/Left Leg [1/0]/1 -> Friction Compensation/1(Right/Left [1/0])
  Product/1 -> Sum1/2
  Desired Acceleration [rad/s^2] [back front]/1 -> Product/1
  Measured Velocity [rad/s] [back front]/1 -> Sum8/2
  kd/1 -> Sum9/2
  Desired Position [rad] [back front]/1 -> Sum7/1
  Sum8/1 -> kd/1
  Sum9/1 -> Sum1/1
  Measured Position [rad] [back front]/1 -> Sum7/2
  Sum7/1 -> kp/1
  kp/1 -> Sum9/1

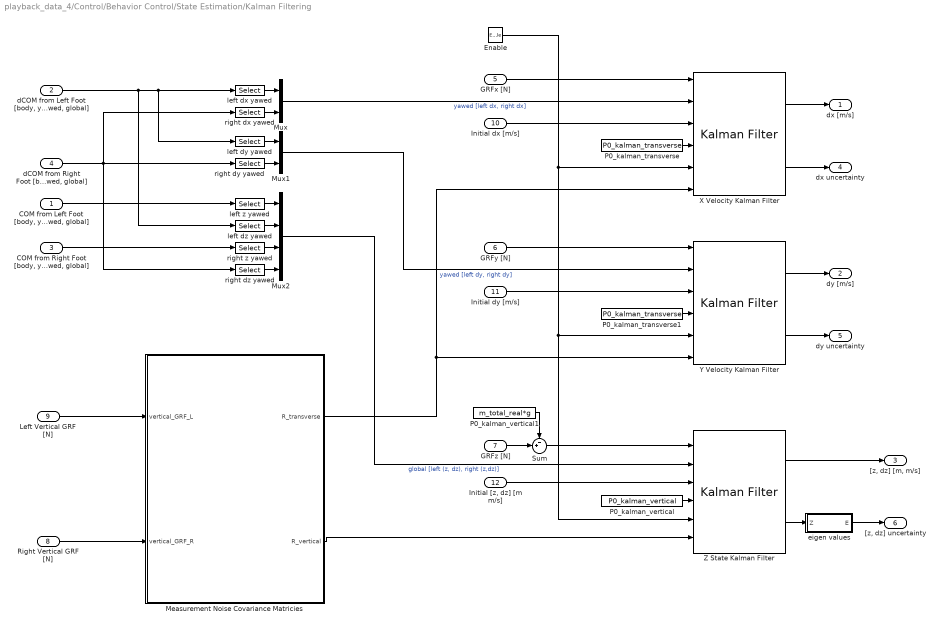
== system playback_data_4/Control/Behavior Control/State Estimation/Kalman Filtering ==
  "COM from Left Foot [body, yawed, global]" : Inport  SampleTime=sample_time
  "dCOM from Left Foot [body, yawed, global]" : Inport  Port=2  SampleTime=sample_time
  "COM from Right Foot [body, yawed, global]" : Inport  Port=3  SampleTime=sample_time
  "dCOM from Right Foot [body, yawed, global]" : Inport  Port=4  SampleTime=sample_time
  GRFx [N] : Inport  Port=5  SampleTime=sample_time
  GRFy [N] : Inport  Port=6  SampleTime=sample_time
  GRFz [N] : Inport  Port=7  SampleTime=sample_time
  Right Vertical GRF [N] : Inport  Port=8  SampleTime=sample_time
  Left Vertical GRF [N] : Inport  Port=9  SampleTime=sample_time
  Initial dx [m/s] : Inport  Port=10  PortDimensions=1  SampleTime=sample_time
  Initial dy [m/s] : Inport  Port=11  PortDimensions=1  SampleTime=sample_time
  "Initial [z, dz] [m m/s]" : Inport  Port=12  PortDimensions=2  SampleTime=sample_time
  Enable : EnablePort  ShowOutputPort=on
  Measurement Noise Covariance Matricies : MATLAB Function  TreatAsAtomicUnit=on
  Mux : Mux  Inputs=2
  Mux1 : Mux  Inputs=2
  Mux2 : Mux
  P0_kalman_transverse : Constant  Value=P0_kalman_transverse
  P0_kalman_transverse1 : Constant  Value=P0_kalman_transverse
  P0_kalman_vertical : Constant  Value=P0_kalman_vertical
  P0_kalman_vertical1 : Constant  Value=m_total_real*g
  Sum : Sum  Inputs=-+|
  X Velocity Kalman Filter : ctrlSharedLib/Kalman Filter  TimeDomain=Discrete-Time  UseCurrentEstimator=on  ModelSource=Individual A, B, C, D matrices  ModelSourceVariable=A_kf  A=A_kalman_transverse  B=B_kalman_transverse  C=C_kalman_transverse  D=0  NumberOfStates=2  NumberOfInputs=1  NumberOfOutputs=2  InitialEstimateSource=Input port  X0=initial_dx_estimate  P0=P0_kalman_transverse  UseK=off  UseGH=on  NumberOfProcessNoiseInputs=1  G=G_kalman_transverse  TimeInvariantG=on  H=0  TimeInvariantH=on  Q=Q_kalman_GRF  TimeInvariantQ=on  R=1  TimeInvariantR=off  N=0  TimeInvariantN=on  AddInputPort=on  AddEnablePort=off  ExternalReset=Either  OutputEstimatedY=off  OutputP=on  Ts=sample_time
  Y Velocity Kalman Filter : ctrlSharedLib/Kalman Filter  TimeDomain=Discrete-Time  UseCurrentEstimator=on  ModelSource=Individual A, B, C, D matrices  ModelSourceVariable=A_kf  A=A_kalman_transverse  B=B_kalman_transverse  C=C_kalman_transverse  D=0  NumberOfStates=2  NumberOfInputs=1  NumberOfOutputs=2  InitialEstimateSource=Input port  X0=initial_dy_estimate  P0=P0_kalman_transverse  UseK=off  UseGH=on  NumberOfProcessNoiseInputs=1  G=G_kalman_transverse  TimeInvariantG=on  H=0  TimeInvariantH=on  Q=Q_kalman_GRF  TimeInvariantQ=on  R=1  TimeInvariantR=off  N=0  TimeInvariantN=on  AddInputPort=on  AddEnablePort=off  ExternalReset=Either  OutputEstimatedY=off  OutputP=on  Ts=sample_time
  Z State Kalman Filter : ctrlSharedLib/Kalman Filter  TimeDomain=Discrete-Time  UseCurrentEstimator=on  ModelSource=Individual A, B, C, D matrices  ModelSourceVariable=A_kf  A=A_kalman_vertical  B=B_kalman_vertical  C=C_kalman_vertical  D=0  NumberOfStates=2  NumberOfInputs=1  NumberOfOutputs=2  InitialEstimateSource=Input port  X0=[initial_z_estimate; initial_dz_estimate]  P0=P0_kalman_vertical  UseK=off  UseGH=on  NumberOfProcessNoiseInputs=1  G=G_kalman_vertical  TimeInvariantG=on  H=0  TimeInvariantH=on  Q=Q_kalman_GRF  TimeInvariantQ=on  R=1  TimeInvariantR=off  N=0  TimeInvariantN=on  AddInputPort=on  AddEnablePort=off  ExternalReset=Either  OutputEstimatedY=off  OutputP=on  Ts=sample_time
  eigen values : MATLAB Function  TreatAsAtomicUnit=on
  left dx yawed : Selector  InputPortWidth=9  Indices=[4]
  left dy yawed : Selector  InputPortWidth=9  Indices=[5]
  left dz yawed : Selector  InputPortWidth=9  Indices=[6]
  left z yawed : Selector  InputPortWidth=9  Indices=[6]
  right dx yawed : Selector  InputPortWidth=9  Indices=[4]
  right dy yawed : Selector  InputPortWidth=9  Indices=[5]
  right dz yawed : Selector  InputPortWidth=9  Indices=[6]
  right z yawed : Selector  InputPortWidth=9  Indices=[6]
  dx [m/s] : Outport
  dy [m/s] : Outport  Port=2
  "[z, dz] [m, m/s]" : Outport  Port=3
  dx uncertainty : Outport  Port=4
  dy uncertainty : Outport  Port=5
  "[z, dz] uncertainty" : Outport  Port=6
  wires:
  eigen values/1(E) -> "[z, dz] uncertainty"/1
  Z State Kalman Filter/2 -> eigen values/1(Z)
  Y Velocity Kalman Filter/2 -> dy uncertainty/1
  X Velocity Kalman Filter/2 -> dx uncertainty/1
  Enable/1 -> X Velocity Kalman Filter/5, Y Velocity Kalman Filter/5, Z State Kalman Filter/5
  P0_kalman_vertical1/1 -> Sum/1
  GRFz [N]/1 -> Sum/2
  "Initial [z, dz] [m m/s]"/1 -> Z State Kalman Filter/3
  P0_kalman_vertical/1 -> Z State Kalman Filter/4
  Initial dy [m/s]/1 -> Y Velocity Kalman Filter/3
  P0_kalman_transverse1/1 -> Y Velocity Kalman Filter/4
  Initial dx [m/s]/1 -> X Velocity Kalman Filter/3
  P0_kalman_transverse/1 -> X Velocity Kalman Filter/4
  "COM from Right Foot [body, yawed, global]"/1 -> right z yawed/1
  "COM from Left Foot [body, yawed, global]"/1 -> left z yawed/1
  right dz yawed/1 -> Mux2/4
  left dz yawed/1 -> Mux2/2
  right z yawed/1 -> Mux2/3
  left z yawed/1 -> Mux2/1
  right dy yawed/1 -> Mux1/2
  left dy yawed/1 -> Mux1/1
  right dx yawed/1 -> Mux/2
  "dCOM from Right Foot [body, yawed, global]"/1 -> right dy yawed/1, right dz yawed/1, right dx yawed/1
  left dx yawed/1 -> Mux/1
  "dCOM from Left Foot [body, yawed, global]"/1 -> left dz yawed/1, left dx yawed/1, left dy yawed/1
  X Velocity Kalman Filter/1 -> dx [m/s]/1
  Y Velocity Kalman Filter/1 -> dy [m/s]/1
  Z State Kalman Filter/1 -> "[z, dz] [m, m/s]"/1
  Left Vertical GRF [N]/1 -> Measurement Noise Covariance Matricies/1(vertical_GRF_L)
  Right Vertical GRF [N]/1 -> Measurement Noise Covariance Matricies/2(vertical_GRF_R)
  Mux/1 -> X Velocity Kalman Filter/2  "yawed [left dx, right dx]"
  Sum/1 -> Z State Kalman Filter/1
  Mux1/1 -> Y Velocity Kalman Filter/2  "yawed [left dy, right dy]"
  Measurement Noise Covariance Matricies/1(R_transverse) -> Y Velocity Kalman Filter/6, X Velocity Kalman Filter/6
  Measurement Noise Covariance Matricies/2(R_vertical) -> Z State Kalman Filter/6
  GRFx [N]/1 -> X Velocity Kalman Filter/1
  Mux2/1 -> Z State Kalman Filter/2  "global [left (z, dz), right (z,dz)]"
  GRFy [N]/1 -> Y Velocity Kalman Filter/1

== system playback_data_4/Control/Subsystem/SEA Controller (Torque)/Antiresonance Compensation ==
  Torque : Inport
  Notch Filter (Flight) : DiscreteTransferFcn  Numerator=[K_notch_f1 K_notch_f1*A1_notch_f1 K_notch_f1*A2_notch_f1]  Denominator=[1 B1_notch_f1 B2_notch_f1]  SampleTime=sample_time
  Filtered Torque : Outport
  wires:
  Notch Filter (Flight)/1 -> Filtered Torque/1
  Torque/1 -> Notch Filter (Flight)/1

== system playback_data_4/Control/Subsystem/SEA Controller (Torque)/Friction Compensation ==
  Motor Velocity [rad/s] : Inport
  Gain2 : Gain  Gain=sea_coulomb_friction_direction_switch_sensitivity
  KdGain2 : Gain  Description=xPCTag(1)=kd_sea_torque;  Gain=sea_coulomb_friction
  Trigonometric Function : Trigonometry  Operator=tanh
  Friction Compensation [Nm] : Outport
  wires:
  Trigonometric Function/1 -> KdGain2/1
  Gain2/1 -> Trigonometric Function/1
  Motor Velocity [rad/s]/1 -> Gain2/1
  KdGain2/1 -> Friction Compensation [Nm]/1

== system playback_data_4/Control/Subsystem/SEA Controller (Torque)/Loaded Unloaded Switch ==
  Loaded Signal : Inport
  Unloaded Signal : Inport  Port=2
  Loaded/Unloaded [1/0] x4 : Inport  Port=3
  Demux : Demux
  Demux1 : Demux
  Demux2 : Demux
  Mux : Mux
  Switch{,1..3} (4 alike) : Switch  Criteria=u2 ~= 0
  Signal : Outport
  wires:
  Demux2/1 -> Switch/3
  Demux2/2 -> Switch1/3
  Demux2/3 -> Switch2/3
  Demux2/4 -> Switch3/3
  Unloaded Signal/1 -> Demux2/1
  Demux1/4 -> Switch3/1
  Demux1/3 -> Switch2/1
  Demux1/2 -> Switch1/1
  Demux1/1 -> Switch/1
  Loaded Signal/1 -> Demux1/1
  Demux/1 -> Switch/2
  Switch/1 -> Mux/1
  Mux/1 -> Signal/1
  Loaded/Unloaded [1/0] x4/1 -> Demux/1
  Switch3/1 -> Mux/4
  Switch2/1 -> Mux/3
  Switch1/1 -> Mux/2
  Demux/2 -> Switch1/2
  Demux/3 -> Switch2/2
  Demux/4 -> Switch3/2

== system playback_data_4/Control/Subsystem/SEA Controller (Torque)/critical damping ==
  p gain : Inport
  Gain : Gain  Gain=0.9
  Gain1 : Gain  Gain=2
  Gain2 : Gain  Gain=j_motor
  Spring Stiffness1 : Gain  Gain=1./k_sea
  Sqrt : Sqrt  SaturateOnIntegerOverflow=on
  d gain : Outport
  wires:
  p gain/1 -> Spring Stiffness1/1
  Gain/1 -> Gain1/1
  Sqrt/1 -> Gain/1
  Gain2/1 -> Sqrt/1
  Spring Stiffness1/1 -> Gain2/1
  Gain1/1 -> d gain/1

== system playback_data_4/Control/Behavior Control/Primary and Lateral Behavior/Circular Buffer/Enabled on Touchdown ==
  In : Inport
  Enable : EnablePort
  Out : Outport
  wires:
  In/1 -> Out/1

== system playback_data_4/Control/Behavior Control/Primary and Lateral Behavior/Flight/Back//Front Motor PD ==
  Desired Position [rad] [back front] : Inport
  Desired Velocity [rad/s] [back front] : Inport  Port=2
  Desired Acceleration [rad/s^2] [back front] : Inport  Port=3
  Measured Position [rad] [back front] : Inport  Port=4
  Measured Velocity [rad/s] [back front] : Inport  Port=5
  Right/Left Leg [1/0] : Inport  Port=6
  Divide : Product  Inputs=*/
  Friction Compensation : Subsystem
  Load Torque in Flight : Constant  Value=30
  Motor Efficiency : MATLAB Function  TreatAsAtomicUnit=on
  Product : Product
  RadPerSecToRotorRpm : Gain  Gain=60*LEG_MTR_GEAR_RATIO/(2*pi)
  Sum1 : Sum  Inputs=|++
  Sum2 : Sum  Inputs=|++
  Sum7 : Sum  Inputs=|+-
  Sum8 : Sum  Inputs=|+-
  Sum9 : Sum
  kd : Gain  Gain=kd_motor
  kp : Gain  Gain=kp_motor
  reflected inertia : Constant  Value=j_motor
  Commanded Torque [Nm] [back front] : Outport
  wires:
  Load Torque in Flight/1 -> Motor Efficiency/2(load_torque)
  Sum1/1 -> Divide/1
  Divide/1 -> Sum2/1
  Motor Efficiency/1(mu) -> Divide/2
  RadPerSecToRotorRpm/1 -> Motor Efficiency/1(rpm)
  Friction Compensation/1(Friction Compensation [Nm]) -> Sum2/2
  reflected inertia/1 -> Product/2
  Desired Velocity [rad/s] [back front]/1 -> Sum8/1, Friction Compensation/2(Commanded Velocity [rad/s] [back front]), RadPerSecToRotorRpm/1
  Sum2/1 -> Commanded Torque [Nm] [back front]/1
  Right/Left Leg [1/0]/1 -> Friction Compensation/1(Right/Left [1/0])
  Product/1 -> Sum1/2
  Desired Acceleration [rad/s^2] [back front]/1 -> Product/1
  Measured Velocity [rad/s] [back front]/1 -> Sum8/2
  kd/1 -> Sum9/2
  Desired Position [rad] [back front]/1 -> Sum7/1
  Sum8/1 -> kd/1
  Sum9/1 -> Sum1/1
  Measured Position [rad] [back front]/1 -> Sum7/2
  Sum7/1 -> kp/1
  kp/1 -> Sum9/1

== system playback_data_4/Control/Behavior Control/Primary and Lateral Behavior/Flight/Hold Values on Takeoff ==
  in : Inport
  Trigger : TriggerPort  ShowOutputPort=on  PortDimensions=1
  Subsystem : Subsystem
  out : Outport
  wires:
  in/1 -> Subsystem/1(in)
  Subsystem/1(out) -> out/1
  Trigger/1 -> Subsystem/Enable

== system playback_data_4/Control/Behavior Control/Primary and Lateral Behavior/Stance/Hold Values on Takeoff ==
  in : Inport
  Trigger : TriggerPort  ShowOutputPort=on  PortDimensions=1
  Subsystem : Subsystem
  out : Outport
  wires:
  in/1 -> Subsystem/1(in)
  Subsystem/1(out) -> out/1
  Trigger/1 -> Subsystem/Enable

== system playback_data_4/Control/Behavior Control/Primary and Lateral Behavior/Stance/Hold Values on Touchdown ==
  in : Inport
  Trigger : TriggerPort  ShowOutputPort=on  PortDimensions=1
  Subsystem : Subsystem
  out : Outport
  wires:
  Trigger/1 -> Subsystem/Enable
  Subsystem/1(out) -> out/1
  in/1 -> Subsystem/1(in)

== system playback_data_4/Control/Behavior Control/Secondary Leg Behavior/Back//Front Motor PD/Friction Compensation ==
  Right/Left [1/0] : Inport
  Commanded Velocity [rad/s] [back front] : Inport  Port=2
  Product : Product
  Sign : Signum
  Sum1 : Sum
  Switch : Switch  Criteria=u2 ~= 0
  Switch1 : Switch  Criteria=u2 ~= 0
  coulomb_friction_left : Constant  Value=sea_coulomb_friction(3:4)
  coulomb_friction_right : Constant  Value=sea_coulomb_friction(1:2)
  offset_friction_left : Constant  Value=sea_offset_friction(3:4)
  offset_friction_right : Constant  Value=sea_offset_friction(1:2)
  Friction Compensation [Nm] : Outport
  wires:
  Sign/1 -> Product/1
  Switch1/1 -> Product/2
  coulomb_friction_left/1 -> Switch1/3
  coulomb_friction_right/1 -> Switch1/1
  offset_friction_left/1 -> Switch/3
  offset_friction_right/1 -> Switch/1
  Right/Left [1/0]/1 -> Switch/2, Switch1/2
  Product/1 -> Sum1/1
  Sum1/1 -> Friction Compensation [Nm]/1
  Switch/1 -> Sum1/2
  Commanded Velocity [rad/s] [back front]/1 -> Sign/1

== system playback_data_4/Control/Behavior Control/Primary and Lateral Behavior/Flight/Back//Front Motor PD/Friction Compensation ==
  Right/Left [1/0] : Inport
  Commanded Velocity [rad/s] [back front] : Inport  Port=2
  Product : Product
  Sign : Signum
  Sum1 : Sum
  Switch : Switch  Criteria=u2 ~= 0
  Switch1 : Switch  Criteria=u2 ~= 0
  coulomb_friction_left : Constant  Value=sea_coulomb_friction(3:4)
  coulomb_friction_right : Constant  Value=sea_coulomb_friction(1:2)
  offset_friction_left : Constant  Value=sea_offset_friction(3:4)
  offset_friction_right : Constant  Value=sea_offset_friction(1:2)
  Friction Compensation [Nm] : Outport
  wires:
  Sign/1 -> Product/1
  Switch1/1 -> Product/2
  coulomb_friction_left/1 -> Switch1/3
  coulomb_friction_right/1 -> Switch1/1
  offset_friction_left/1 -> Switch/3
  offset_friction_right/1 -> Switch/1
  Right/Left [1/0]/1 -> Switch/2, Switch1/2
  Product/1 -> Sum1/1
  Sum1/1 -> Friction Compensation [Nm]/1
  Switch/1 -> Sum1/2
  Commanded Velocity [rad/s] [back front]/1 -> Sign/1

== system playback_data_4/Control/Behavior Control/Primary and Lateral Behavior/Flight/Hold Values on Takeoff/Subsystem ==
  in : Inport
  Enable : EnablePort
  out : Outport
  wires:
  in/1 -> out/1

== system playback_data_4/Control/Behavior Control/Primary and Lateral Behavior/Stance/Hold Values on Takeoff/Subsystem ==
  in : Inport
  Enable : EnablePort
  out : Outport
  wires:
  in/1 -> out/1

== system playback_data_4/Control/Behavior Control/Primary and Lateral Behavior/Stance/Hold Values on Touchdown/Subsystem ==
  in : Inport
  Enable : EnablePort
  out : Outport
  wires:
  in/1 -> out/1

== stateflow chart playback_data_4/Control/Behavior Control/Contact State Machine/State Machine ==
  state TouchDown
  state LockedContact
  state Unloading
  state Takeoff
  state Flight
  (junction 91) -> TouchDown
  TouchDown -> (junction 130) [order 2] : [vertical_grf < contact_threshold]
  (junction 93) -> (junction 91)
  (junction 130) -> (junction 128)
  TouchDown -> LockedContact [order 1] : [vertical_grf > loaded_threshold]
  (junction 115) -> LockedContact
  (junction 118) -> (junction 115)
  LockedContact -> Unloading : [z_velocity >= 0 && previous_z_velocity < 0]
  Unloading -> LockedContact [order 2] : [vertical_grf > loaded_threshold && z_velocity < 0]
  (junction 122) -> (junction 118)
  Unloading -> Takeoff [order 1] : [vertical_grf < contact_threshold]
  Takeoff -> Flight : after(t_flight,sec)
  (default) -> Flight
  Flight -> (junction 93) : [vertical_grf > contact_threshold]
  (junction 128) -> Flight
  data: z_velocity input; previous_z_velocity input; vertical_grf input; t_flight parameter; max_leg_length parameter; contact_threshold parameter; loaded_threshold parameter; TouchDown output boolean; LockedContact output boolean; Unloading output boolean; Takeoff output boolean; Flight output boolean

== matlab function playback_data_4/Control/Behavior Control/Primary and Lateral Behavior/Stance/LQR Feedback for Desired Forward GRF ==
  data: hopping input; stance input; GRFx_desired output; netural_pitch_ff output; true_ff output; GRFx_lqr output; ddtheta_star output; ddtheta_star_neutral output; xdx input; thetadtheta input; zdz input; Fz input; xdx_ref input size=2; theta_star input; K_sag input; P_sag input; measured_GRF input; i_robot parameter; cost_to_go output double size=1; ang_mom output; desired_standing_torso_pitch parameter; k_LQR_sagittal_infinite parameter; P_LQR_sagittal_infinite parameter
%% LQR for x state

% stance: 1 if in stance, 0 otherwise
% xdx: [ x from stance leg to COM, dx of COM]
% thetadtheta: [pitch, dpitch]
% zdz: [z of COM, dz of COM]
% Fz: Desired z GRF
% xdx_ref: [x, dx] current reference point for COM
% theta_star: desired torso pitch
% K_sag: time dependent LQR gain


% sagittal_state: [x, pitch, dx, dptich]
% theta_star: desired torso pitch


function [GRFx_desired, netural_pitch_ff, true_ff, GRFx_lqr, ddtheta_star, ddtheta_star_neutral, cost_to_go, ang_mom]  =  ...
    LQR_Sagittal(hopping, stance, xdx, thetadtheta, zdz, Fz, xdx_ref, theta_star, K_sag, P_sag, measured_GRF, i_robot,...
    desired_standing_torso_pitch, k_LQR_sagittal_infinite, P_LQR_sagittal_infinite)


    sagittal_state = [xdx(1); thetadtheta(1); xdx(2); thetadtheta(2)];
    netural_pitch_ff = Fz*xdx(1)/zdz(1);
    true_ff = Fz*xdx_ref(1)/zdz(1);
    
    if hopping
        sagittal_reference = [xdx_ref(1), theta_star, xdx_ref(2), 0]';
        sagittal_error = (sagittal_state - sagittal_reference);
        cost_to_go = 0.5*sagittal_error'*P_sag*sagittal_error;
        GRFx_lqr = - K_sag*sagittal_error;
        GRFx_desired = true_ff + GRFx_lqr;
    else
        sagittal_reference = [xdx_ref(1), desired_standing_torso_pitch, xdx_ref(2), 0]';
        sagittal_error = (sagittal_state - sagittal_reference);
        cost_to_go = 0.5*sagittal_error'*P_LQR_sagittal_infinite*sagittal_error;
        %GRFx_desired = i_robot/zdz(1)*(150*(thetadtheta(1)-desired_standing_torso_pitch) + 30*thetadtheta(2)) + netural_pitch_ff;
        GRFx_lqr = - k_LQR_sagittal_infinite*sagittal_error;
        GRFx_desired = GRFx_lqr;
    end

    GRFx_desired = min(max(GRFx_desired, -0.5*abs(measured_GRF(3))), 0.5*abs(measured_GRF(3))); % saturate to friction cone
    
    if stance == 0
      GRFx_lqr = 0;
      cost_to_go = 0;
      netural_pitch_ff = 0;
      true_ff = 0;
    end
    
    % quantities for logging
    ddtheta_star_neutral = -(GRFx_lqr)*zdz(1)/i_robot;
    ddtheta_star = -(GRFx_desired - netural_pitch_ff)*zdz(1)/i_robot;
    ang_mom = i_robot*thetadtheta(2);
end

== matlab function playback_data_4/Control/Behavior Control/Torque Distribution Right/Motor Torque Saturation Optimization ==
  data: x1s input; t1 output; x2s input; lambda1 parameter; lambda2 parameter; max_torque_sagittal parameter; t2 output
% Optimal leg motor torque distribution
function [t1, t2] = distribute_torque(x1s, x2s, lambda1, lambda2, max_torque_sagittal)

s = max_torque_sagittal;

% possible solutions
x1 = [                                                      x1s;
                                                            0;
                                                            s;
                                                            0;
                                                           -s;
  (lambda2*s + lambda1*x1s - lambda2*x2s)/(lambda1 + lambda2);
  (lambda1*x1s - lambda2*s + lambda2*x2s)/(lambda1 + lambda2);
  (lambda2*s + lambda1*x1s + lambda2*x2s)/(lambda1 + lambda2);
 -(lambda2*s - lambda1*x1s + lambda2*x2s)/(lambda1 + lambda2)];
 
x2 = [                                                      x2s;
                                                            s;
                                                            0;
                                                           -s;
                                                            0;
  (lambda1*s - lambda1*x1s + lambda2*x2s)/(lambda1 + lambda2);
  (lambda1*s + lambda1*x1s + lambda2*x2s)/(lambda1 + lambda2);
  (lambda1*x1s - lambda1*s + lambda2*x2s)/(lambda1 + lambda2);
 -(lambda1*s + lambda1*x1s - lambda2*x2s)/(lambda1 + lambda2)];

% test constraints
c1 = s - x1 - x2 >= 0;
c2 = s + x1 + x2 >= 0;
c3 = s - x1 + x2 >= 0;
c4 = s + x1 - x2 >= 0;
constraints = c1 & c2 & c3 & c4;

% objective function to maximize
f = -lambda1*(x1-x1s).^2-lambda2*(x2-x2s).^2;
satisfied = find(constraints);
[~,I] = max(f(satisfied));

t1 = x1(satisfied(I));
t2 = x2(satisfied(I));
